simulink model "Lab1_kalman_real"  (R2018a)
settings: Solver=VariableStepAuto  StartTime=0.0  StopTime=1000  RelTol=1e-3
values from neighbouring files (symbols this model uses):
  Ak = [0.998215417622  0; 0.00178298906287  0.998215417622]    [LabB_FInal_version2.mat]
  Bk = [0.00151379915633 1.35155387491e-06]    [LabB_FInal_version2.mat]
  C1 = [1 0]    [Lab1.m]    (also in LabB_FInal_version2.mat; Untitled.m)
  C2 = [0 1]    [Lab1.m]    (also in LabB_FInal_version2.mat; Untitled.m)
  Ck = [0 1]    [LabB_FInal_version2.mat]
  h = 5:1:15    [Lab1.m]    (also in LabB_FInal_version2.mat = [3 4 5 6 7 8 9 10 11 12 13 14 ... (13 elements, 1x13)]; Untitled.m = 3:1:15)
  hV = [1.826, 2.539, 3.452, 4.18, 4.99, 5.762, 6.665, 7.36, 8.193, 8.93, 9.66]    [Lab1.m]    (also in LabB_FInal_version2.mat = [0.68 1.53 2.27 3.07 3.82 4.63 5.33 6.14 6.89 7.56 8.38 9.19; Untitled.m = [.68 1.53 2.27 3.07 3.82 4.63 5.33 6.14 6.89 7.56 8.38 9.19 )
  K = K'    [Lab1.m]    (also in LabB_FInal_version2.mat = [5.99248777663 0.992989193414]; Untitled.m)
  v = 1:1:10    [Lab1.m]    (also in LabB_FInal_version2.mat = [1 2 3 4 5 6 7 8 9 10]; Untitled.m)
  vt = [21.18, 26.66 30.97, 34.28, 37.92, 39.73, 42.53, 45.45, 46.49, 47.67]    [Lab1.m]    (also in LabB_FInal_version2.mat = [21.18 26.66 30.97 34.28 37.92 39.73 42.53 45.45 46.49 47.67; Untitled.m)
undefined symbols (not defined in the file or in its folder): National_Instruments, PCI
libraries: sldrtlib x2
settings Model: Creator=scofre-5  LastModifiedBy=scofre-5

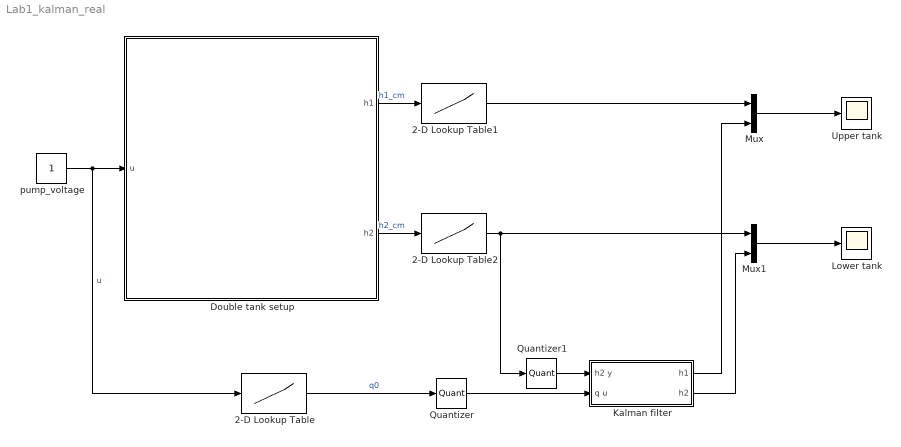
== system Lab1_kalman_real ==
  2-D Lookup Table : Lookup_n-D  NumberOfTableDimensions=1  BreakpointsForDimension1=x  BreakpointsForDimension2=[1:3]  Table=y  RndMeth=Simplest  InputSameDT=on  mask{x=v, y=vt}
      mask prompts: x "Values on x-axis"; y "Values on y-axis"
  2-D Lookup Table1 : Lookup_n-D  NumberOfTableDimensions=1  BreakpointsForDimension1=x  BreakpointsForDimension2=[1:3]  Table=y  RndMeth=Simplest  InputSameDT=on  mask{x=hV, y=h}
      mask prompts: x "Values on x-axis"; y "Values on y-axis"
  2-D Lookup Table2 : Lookup_n-D  NumberOfTableDimensions=1  BreakpointsForDimension1=x  BreakpointsForDimension2=[1:3]  Table=y  RndMeth=Simplest  InputSameDT=on  mask{x=hV, y=h}
      mask prompts: x "Values on x-axis"; y "Values on y-axis"
  Double tank setup : Subsystem  AncestorBlock=R0002E_lib/Double tank setup  StopFcn=|  mask(Realtime interface for the tank process){ts=0.02, h1_ch=0, h2_ch=1, u_ch=0}
      | chn =get_param(gcb,'u_ch');                          
      | s = daq.createSession('ni');                         
      | channel = ['ao',chn];                                
      | s.addAnalogOutputChannel('Dev1', channel, 'Voltage');
      | x = zeros(5,1);                                      
      | s.queueOutputData(x);                                
      | lh = s.addlistener('DataRequired', ...               
      | @(src,event) src.queueOutputData(x));                
      | s.startBackground();                                 
      | s.wait();                                            
      | s.stop();                                            
      | delete(lh);                                          
      | clear chn;                                           
      | clear s;                                             
      | clear channel;                                       
      | clear lh;                                            
      | clear x;
      mask prompts: ts "Sample time"; h1_ch "A/D Channel for upper tank"; h2_ch "A/D Channel for lower tank"; u_ch "D/A Channel for pump"
      mask help:
      | This block represents the physical interface from the computer to the tank process.
      |
      | The input u is the voltage that is provided for the pump, the output h1 is the measured level in the upper tank in [V] and the output h2 is the
      | measured level in the lower tank in [V].
      |
      | You need to provide the sample rate at which the voltage to the pump is updated and the level measurements are sampled. The sample rate should not be less than 0.02 seconds.
      mask Display:
      | x=363;
      | y=381;
      | image(imread('tank_icon.jpg'));
      | text(250/x,309/y,'Sensor');
      | text(260/x,169/y,'Sensor');
      | text(335/x,289/y,'A');
      | text(351/x,283/y,'D');
      | text(335/x,100/y,'A');
      | text(351/x,95/y,'D');
      | text(22/x,187/y,'A');
      | text(5/x,195/y,'D');
      | text(225/x,278/y,'h_1','texmode','on');
      | text(225/x,146/y,'h_2','texmode','on');
      | text(300/x,270/y,sprintf('AI-%d',h1_ch));
      | text(300/x,80/y,sprintf('AI-%d',h2_ch));
      | text(40/x,173/y,sprintf('AO-%d',u_ch));
  Kalman filter : Subsystem
  Lower tank : Scope
  Mux : Mux  Inputs=2
  Mux1 : Mux  Inputs=2
  Quantizer : Quantizer  QuantizationInterval=0.005
  Quantizer1 : Quantizer  QuantizationInterval=0.005
  Upper tank : Scope
  pump_voltage : Constant
  wires:
  Mux/1 -> Upper tank/1
  Double tank setup/1(h1) -> 2-D Lookup Table1/1  "h1_cm"
  Kalman filter/1(h1) -> Mux/2
  Quantizer1/1 -> Kalman filter/1("h2 y ")
  pump_voltage/1 -> Double tank setup/1(u), 2-D Lookup Table/1  "u"
  Double tank setup/2(h2) -> 2-D Lookup Table2/1  "h2_cm"
  2-D Lookup Table/1 -> Quantizer/1  "q0"
  Quantizer/1 -> Kalman filter/2(q u)
  Mux1/1 -> Lower tank/1
  2-D Lookup Table1/1 -> Mux/1
  2-D Lookup Table2/1 -> Mux1/1, Quantizer1/1
  Kalman filter/2("h2 ") -> Mux1/2

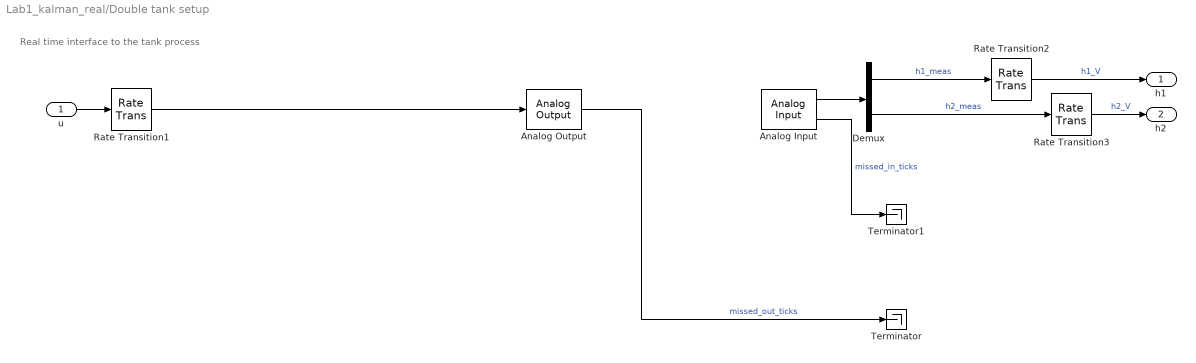
== system Lab1_kalman_real/Double tank setup ==
  note: Real time interface to the tank process
  u : Inport
  Analog Input : sldrtlib/Analog Input  SampleTime=ts  MaxMissedTicks=500000000  ShowMissedTicks=on  YieldWhenWaiting=off  DrvName=National_Instruments/PCI-6024E  DrvAddress=4294967295  DrvOptions=[0 0 0 0 0 0]  Channels=[h1_ch+1,h2_ch+1]  RangeMode=1  VoltRange=1  DataType=1
      settings: AttributesFormatString=National Instruments\nPCI-6024E [auto]  SourceProductName=Simulink Desktop Real-Time
  Analog Output : sldrtlib/Analog Output  SampleTime=ts  MaxMissedTicks=500000000  ShowMissedTicks=on  YieldWhenWaiting=off  DrvName=National_Instruments/PCI-6024E  DrvAddress=4294967295  DrvOptions=[0 0 0 0 0 0]  Channels=u_ch+1  RangeMode=1  VoltRange=1  InitialValue=0  FinalValue=0
      settings: AttributesFormatString=National Instruments\nPCI-6024E [auto]  SourceProductName=Simulink Desktop Real-Time
  Demux : Demux  Outputs=2
  Rate Transition1 : RateTransition  OutPortSampleTime=ts
  Rate Transition2 : RateTransition
  Rate Transition3 : RateTransition
  Terminator : Terminator
  Terminator1 : Terminator
  h1 : Outport
  h2 : Outport  Port=2
  wires:
  Rate Transition1/1 -> Analog Output/1
  Rate Transition3/1 -> h2/1  "h2_V"
  Rate Transition2/1 -> h1/1  "h1_V"
  Analog Input/2 -> Terminator1/1  "missed_in_ticks"
  Demux/2 -> Rate Transition3/1  "h2_meas"
  Demux/1 -> Rate Transition2/1  "h1_meas"
  Analog Input/1 -> Demux/1
  Analog Output/1 -> Terminator/1  "missed_out_ticks"
  u/1 -> Rate Transition1/1

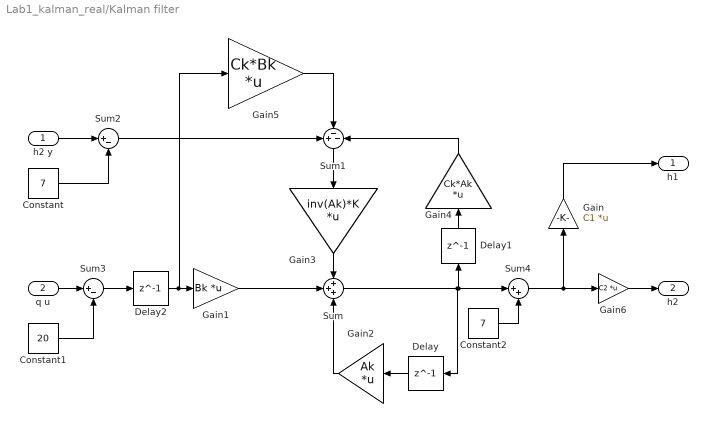
== system Lab1_kalman_real/Kalman filter ==
  "h2 y " : Inport
  q u : Inport  Port=2
  Constant : Constant  Value=7
  Constant1 : Constant  Value=20
  Constant2 : Constant  Value=7
  Delay : Delay  DelayLength=1  InitialCondition=0
  Delay1 : Delay  DelayLength=1  InitialCondition=0
  Delay2 : Delay  DelayLength=1  InitialCondition=0
  Gain : Gain  Gain=C1  Multiplication=Matrix(K*u)
  Gain1 : Gain  Gain=Bk  Multiplication=Matrix(K*u)
  Gain2 : Gain  Gain=Ak  Multiplication=Matrix(K*u)
  Gain3 : Gain  Gain=inv(Ak)*K  Multiplication=Matrix(K*u)
  Gain4 : Gain  Gain=Ck*Ak  Multiplication=Matrix(K*u)
  Gain5 : Gain  Gain=Ck*Bk  Multiplication=Matrix(K*u)
  Gain6 : Gain  Gain=C2  Multiplication=Matrix(K*u)
  Sum : Sum  Inputs=+++
  Sum1 : Sum  Inputs=+--
  Sum2 : Sum  Inputs=|+-
  Sum3 : Sum  Inputs=|+-
  Sum4 : Sum  Inputs=|++
  h1 : Outport
  "h2 " : Outport  Port=2
  wires:
  Gain5/1 -> Sum1/2
  Gain3/1 -> Sum/1
  Sum/1 -> Sum4/1, Delay1/1, Delay/1
  Delay2/1 -> Gain5/1, Gain1/1
  Gain4/1 -> Sum1/3
  Delay1/1 -> Gain4/1
  Gain1/1 -> Sum/2
  Sum1/1 -> Gain3/1
  Delay/1 -> Gain2/1
  Gain2/1 -> Sum/3
  "h2 y "/1 -> Sum2/1
  Sum2/1 -> Sum1/1
  Constant/1 -> Sum2/2
  q u/1 -> Sum3/1
  Sum3/1 -> Delay2/1
  Constant1/1 -> Sum3/2
  Sum4/1 -> Gain/1, Gain6/1
  Constant2/1 -> Sum4/2
  Gain/1 -> h1/1
  Gain6/1 -> "h2 "/1
